simulink model "csu_lak_linear_accel_kinematics_hrn"  (R2014b)
settings: Solver=FixedStepDiscrete  StartTime=t0  StopTime=tFinal  FixedStep=sim_dt  RelTol=1e-3
libraries: csu_lak_linear_accel_kinematics_lib x1, util_quat_lib x1
settings Model: Creator=escrane  LastModifiedBy=mstewart
settings DebuggingCC: UnderspecifiedInitializationDetection=Classic  MergeDetectMultiDrivingBlocksExec=none

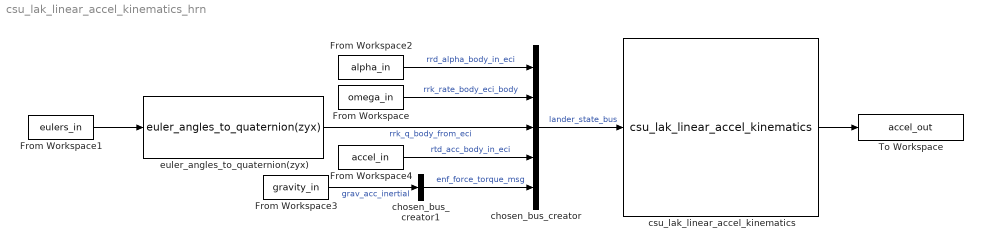
== system csu_lak_linear_accel_kinematics_hrn ==
  From Workspace : FromWorkspace  VariableName=omega_in  SampleTime=0
  From Workspace1 : FromWorkspace  VariableName=eulers_in  SampleTime=0
  From Workspace2 : FromWorkspace  VariableName=alpha_in  SampleTime=0
  From Workspace3 : FromWorkspace  VariableName=gravity_in  SampleTime=0
  From Workspace4 : FromWorkspace  VariableName=accel_in  SampleTime=0
  To Workspace : ToWorkspace  VariableName=accel_out  SaveFormat=Timeseries  SampleTime=-1
  chosen_bus_creator : BusCreator  Inputs=5
  chosen_bus_creator1 : BusCreator  Inputs=1
  csu_lak_linear_accel_kinematics : csu_lak_linear_accel_kinematics_lib/csu_lak_linear_accel_kinematics  accel_position=[0.3 -0.3 0.2]  accel_axis_body_frame_1=[1 0 0]  accel_axis_body_frame_2=[0 0 1]
  euler_angles_to_quaternion(zyx) : util_quat_lib/euler_angles_to_quaternion(zyx)  SystemSampleTime=-1
  wires:
  csu_lak_linear_accel_kinematics/1 -> To Workspace/1
  From Workspace1/1 -> euler_angles_to_quaternion(zyx)/1
  chosen_bus_creator/1 -> csu_lak_linear_accel_kinematics/1  "lander_state_bus"
  From Workspace2/1 -> chosen_bus_creator/1  "rrd_alpha_body_in_eci"
  From Workspace/1 -> chosen_bus_creator/2  "rrk_rate_body_eci_body"
  euler_angles_to_quaternion(zyx)/1 -> chosen_bus_creator/3  "rrk_q_body_from_eci"
  From Workspace4/1 -> chosen_bus_creator/4  "rtd_acc_body_in_eci"
  From Workspace3/1 -> chosen_bus_creator1/1  "grav_acc_inertial"
  chosen_bus_creator1/1 -> chosen_bus_creator/5  "enf_force_torque_msg"
